simulink model "sensor_block"  (Simulink 7.4)
settings: Solver=FixedStepDiscrete  StartTime=0  StopTime=inf  FixedStep=0.05  RelTol=1e-3
settings Model: Creator=kthwsnt  LastModifiedBy=aitorhh
settings SolverCC: PositivePriorityOrder=on
settings DataIOCC: SaveOutput=off  SignalLogging=off  SaveTime=off
settings OptimizationCC: InitFltsAndDblsToZero=on
settings SimEventsCC: propDiagAttribOutput=1  propDiagFcnCallOutput=1  propDiagStatOutput=0

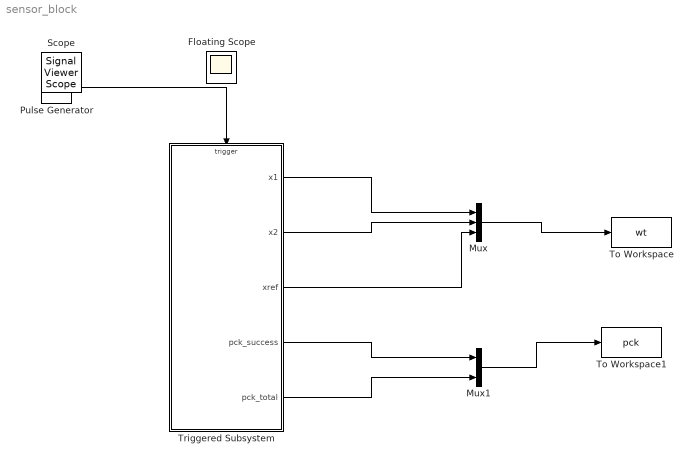
== system sensor_block ==
  Mux : Mux  Inputs=3
  Mux1 : Mux  Inputs=2
  Pulse Generator : DiscretePulseGenerator  PulseType=Time based  Amplitude=1  Period=1  PulseWidth=5  PhaseDelay=0  SampleTime=1
  To Workspace : ToWorkspace  VariableName=wt  SampleTime=-1  SaveFormat=Structure
  To Workspace1 : ToWorkspace  VariableName=pck  SampleTime=-1  SaveFormat=Structure
  Triggered Subsystem : Subsystem  TreatAsAtomicUnit=on
  Floating Scope : Scope
      settings: Floating=on  YMin=10  YMax=10
  Scope : SignalViewerScope  IOType=viewer  RefreshTime=0.035000
      settings: YMin=4660  YMax=4660
  wires:
  Pulse Generator/1 -> Triggered Subsystem/Trigger
  Triggered Subsystem/1(x1) -> Mux/1
  Triggered Subsystem/2(x2) -> Mux/2
  Triggered Subsystem/3(xref) -> Mux/3
  Mux/1 -> To Workspace/1
  Triggered Subsystem/4(pck_success) -> Mux1/1
  Triggered Subsystem/5(pck_total) -> Mux1/2
  Mux1/1 -> To Workspace1/1

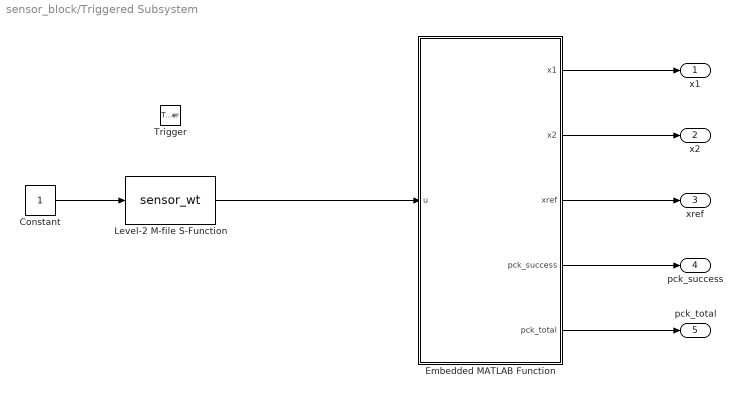
== system sensor_block/Triggered Subsystem ==
  Trigger : TriggerPort
  Constant : Constant  OutDataType=fixdt(1, 16)  OutScaling=2^0
  Embedded MATLAB Function : Stateflow chart
  Level-2 M-file S-Function : M-S-Function  FunctionName=sensor_wt
  x1 : Outport  OutDataType=sfix(16)  OutScaling=2^0
  x2 : Outport  Port=2  OutDataType=sfix(16)  OutScaling=2^0
  xref : Outport  Port=3  OutDataType=sfix(16)  OutScaling=2^0
  pck_success : Outport  Port=4  OutDataType=sfix(16)  OutScaling=2^0
  pck_total : Outport  Port=5  OutDataType=sfix(16)  OutScaling=2^0
  wires:
  Constant/1 -> Level-2 M-file S-Function/1
  Level-2 M-file S-Function/1 -> Embedded MATLAB Function/1(u)
  Embedded MATLAB Function/1(x1) -> x1/1
  Embedded MATLAB Function/2(x2) -> x2/1
  Embedded MATLAB Function/5(pck_total) -> pck_total/1
  Embedded MATLAB Function/4(pck_success) -> pck_success/1
  Embedded MATLAB Function/3(xref) -> xref/1

== matlab function Triggered Subsystem/Embedded MATLAB Function ==
  data: x1 output double; x2 output double; xref output double; u input double; pck_success output double; pck_total output double
function [x1, x2, xref, pck_success, pck_total] = parsePacket(u)
persistent x_ref_vector sample_interval idx


x_ref_vector = [10 10 15 20 12.5 5 0 0];
sample_interval = 500;

if isempty(idx)
    idx = 1;
end
% 02    0f     61 88   e7     34 12     03 00      00 00    00 13    04 e3    0f ff    69    c9     00        c0  2d  40  58 
% 02    0f     61 88   d2     34 12     03 00      00 00    00 00    00 00    07 ff    69    c2     84        32 8d de 02 
% 02    0f     61 88   be     34 12     03 00      00 00    00 00    00 00    07 ff    67    ca     00        c4 f0 8d 03 

% id| length|        |seqnum|  PANID  | Src adr | Dst addr | xc    | theta  |  u_out  | lqi | rssi| mhrLen | timestamp
%           
%#eml
% 02   0f     61 88    9f     34 12     00 00      02 00     00 00     4b      4b         02 04      6b    c2     00       ba 15 28 00 
% id| length|        |seqnum|  PANID  | Dest adr | Src addr | xc    | success |  total  | timestamp | lqi | rssi| mhrLen | timestamp
%00 ff ff 00 00 0a 00 0a 03 47 03 45 00 3e 00 3d 01 e6 

l=length(u);
%
% packet information
%


%
% Sensors and control voltage
%
% xc_sensor=bitor(bitshift(uint16(u(14)),8), uint16(u(15)))*9.2E-5;
% theta_sensor=bitor(bitshift(uint16(u(12)),8), uint16(u(13))) / 1024.0 * 2 * 3.14159265;
% u_control = bitor(bitshift(uint16(u(16)),8), uint16(u(17)));
% u_control = (u_control / 1638) * 4.8 -6;

% Sensor values
x1 = double(bitor(bitshift(uint16(u(9)),8), double(u(10))));
x2 = double(bitor(bitshift(uint16(u(11)),8), double(u(12))));
xref = x_ref_vector(idx);


pck_total = bitor(bitshift(uint16(u(13)),8), uint16(u(14)));
pck_success = bitor(bitshift(uint16(u(15)),8), uint16(u(16)));
delay = bitor(bitshift(uint16(u(17)),8), uint16(u(18)));

if pck_total == (sample_interval -1) && idx ~= length(x_ref_vector)
    idx = idx+1;
    xref = x_ref_vector(idx);
end
